simulink model "simulink_zadnji_zadatak"  (Simulink 8.1)
settings: Solver=ode45  StartTime=0.0  StopTime=10.0  RelTol=1e-3
libraries: dspvision x2
settings Model: Creator=Petra  LastModifiedBy=Petra
settings DataIOCC: SignalLoggingSaveFormat=Dataset
settings OptimizationCC: ExpressionDepthLimit=128
settings DebuggingCC: FcnCallInpInsideContextMsg=EnableAllAsError
settings GRTTargetCC: CombineOutputUpdateFcns=on  GRTInterface=off

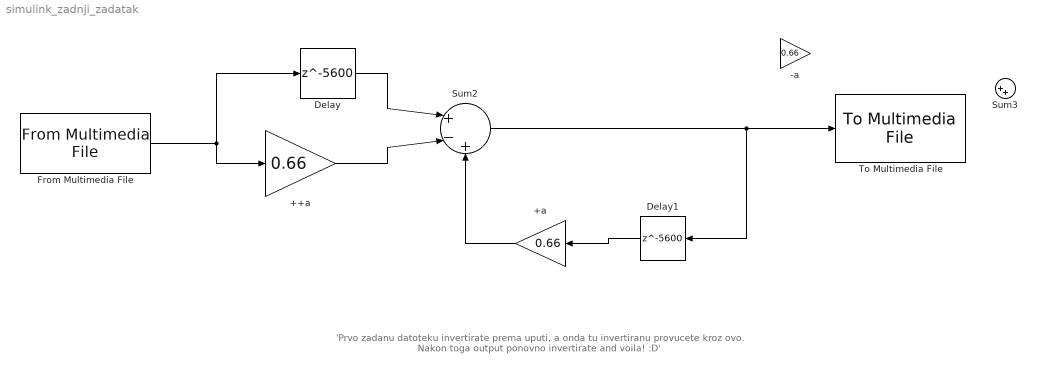
== system simulink_zadnji_zadatak ==
  note: 'Prvo zadanu datoteku invertirate prema uputi, a onda tu invertiranu provucete kroz ovo. Nakon toga output ponovno invertirate and voila! :D'
  ++a : Gain  Gain=0.66
  +a : Gain  Gain=0.66
  "-a " : Gain  Gain=0.66
  Delay : Delay  DelayLength=5600  InputProcessing=Columns as channels (frame based)
  Delay1 : Delay  DelayLength=5600  InputProcessing=Columns as channels (frame based)
  From Multimedia File : dspvision/From Multimedia File  inputFilename=C:\Petra\FER\Obrada Informacija\1. Laboratorijska vjezba\invertirana.wav  loop=on  numPlays=inf  outputStreams=Audio only  videoDataType=single  audioDataType=double  inheritSampleTime=on  userDefinedSampleTime=1/30  noAudioOutput=off  isIntensityVideo=off  fourcc=RGB  colorVideoFormat=Separate color signals  outputEOF=off  dataOrg=Column-major  audioFrameSize=1024  computeAudioFrameSize=off  outSamplingMode=Frame based
  Sum2 : Sum  Inputs=|+-+
  Sum3 : Sum  Inputs=|++
  To Multimedia File : dspvision/To Multimedia File  outputFilename=output.wav  streamSelection=Audio only  videoCompressor=None (uncompressed)  audioCompressor=None (uncompressed)  imagePorts=One multidimensional signal  fileType=WAV  audioDatatype=16-bit integer  fourcc=RGB
  wires:
  Delay/1 -> Sum2/1
  ++a/1 -> Sum2/2
  From Multimedia File/1 -> Delay/1, ++a/1
  +a/1 -> Sum2/3
  Delay1/1 -> +a/1
  Sum2/1 -> Delay1/1, To Multimedia File/1
